simulink model "Manuever_3"  (R2023b)
settings: Solver=FixedStepAuto  StartTime=0.0  StopTime=50  RelTol=1e-3  EnableMultiTasking=on
libraries: legoev3lib x7
settings Model: ExtModeBatchMode=on  ExtModeTrigDuration=2  Creator=Krish  LastModifiedBy=Krish
settings SolverCC: PositivePriorityOrder=on  AutoInsertRateTranBlk=on
settings OptimizationCC: EnhancedBackFolding=on  PassReuseOutputArgsAs=Individual arguments  ZeroExternalMemoryAtStartup=off  ZeroInternalMemoryAtStartup=off  MaxStackSize=64  OptimizeBlockOrder=speed  DifferentSizesBufferReuse=on  OptimizationCustomize=off  EfficientTunableParamExpr=on
settings DebuggingCC: ParameterTunabilityLossMsg=error
settings HardwareCC: ProdBitPerPointer=32  ProdBitPerSizeT=32  ProdBitPerPtrDiffT=32  ProdLargestAtomicInteger=Long  ProdWordSize=32  ProdHWDeviceType=ARM Compatible->ARM 9
settings SFSimCC: MATLABDynamicMemAlloc=off
settings RTWCC: Description=Embedded Coder  SystemTargetFile=ert.tlc  HardwareBoard=LEGO MINDSTORMS EV3  TLCOptions="-aInlineSetEventsForThisBaseRateFcn=TLC_FALSE -aSuppressMultiTaskScheduler=TLC_FALSE  -aRateBasedStepFcn=0"  TemplateMakefile=ert_default_tmf  Toolchain=Sourcery G++ Lite v2009q3
settings CodeAppCC: ForceParamTrailComments=on  IgnoreCustomStorageClasses=off  OperatorAnnotations=on  SimulinkDataObjDesc=on  SFDataObjDesc=on  InsertBlockDesc=on
settings ERTTargetCC: SupportContinuousTime=on  SupportVariableSizeSignals=on  ExtModeTransport=2  ExtModeStaticAlloc=on  ExtModeMexFile=ext_xcp  ExtModeIntrfLevel=Level2 - Open

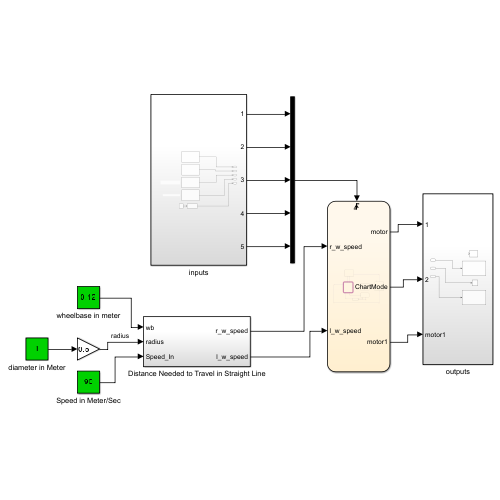
[thumbnail: Simulink's stored preview of the top-level diagram]
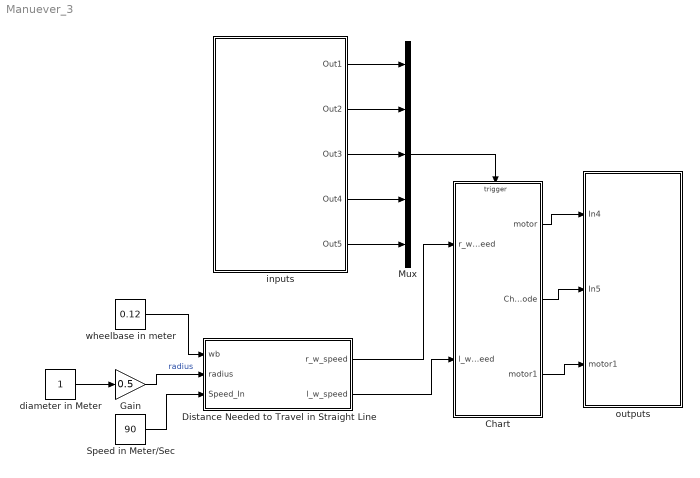
== system Manuever_3 ==
  Chart : Stateflow chart  TreatAsAtomicUnit=on
  Distance Needed to Travel in Straight Line : Subsystem
  Gain : Gain  Gain=0.5
  Mux : Mux  Inputs=5
  Speed in Meter/Sec : Constant  Value=90
  diameter in Meter : Constant
  inputs : Subsystem
  outputs : Subsystem
  wheelbase in meter : Constant  Value=0.12
  wires:
  Mux/1 -> Chart/Trigger
  inputs/1(Out1) -> Mux/1
  inputs/2(Out2) -> Mux/2
  inputs/3(Out3) -> Mux/3
  inputs/4(Out4) -> Mux/4
  inputs/5(Out5) -> Mux/5
  Chart/1(motor) -> outputs/1(In4)
  Chart/2(ChartMode) -> outputs/2(In5)
  Chart/3(motor1) -> outputs/3(motor1)
  Speed in Meter/Sec/1 -> Distance Needed to Travel in Straight Line/3(Speed_In)
  diameter in Meter/1 -> Gain/1
  Distance Needed to Travel in Straight Line/1(r_w_speed) -> Chart/1(r_w_speed)
  wheelbase in meter/1 -> Distance Needed to Travel in Straight Line/1(wb)
  Gain/1 -> Distance Needed to Travel in Straight Line/2(radius)  "radius"
  Distance Needed to Travel in Straight Line/2(l_w_speed) -> Chart/2(l_w_speed)

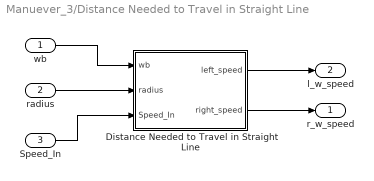
== system Manuever_3/Distance Needed to Travel in Straight Line ==
  wb : Inport
  radius : Inport  Port=2
  Speed_In : Inport  Port=3
  Distance Needed to Travel in Straight Line : Subsystem
  r_w_speed : Outport
  l_w_speed : Outport  Port=2
  wires:
  radius/1 -> Distance Needed to Travel in Straight Line/2(radius)
  Speed_In/1 -> Distance Needed to Travel in Straight Line/3(Speed_In)
  wb/1 -> Distance Needed to Travel in Straight Line/1(wb)
  Distance Needed to Travel in Straight Line/2(right_speed) -> r_w_speed/1
  Distance Needed to Travel in Straight Line/1(left_speed) -> l_w_speed/1

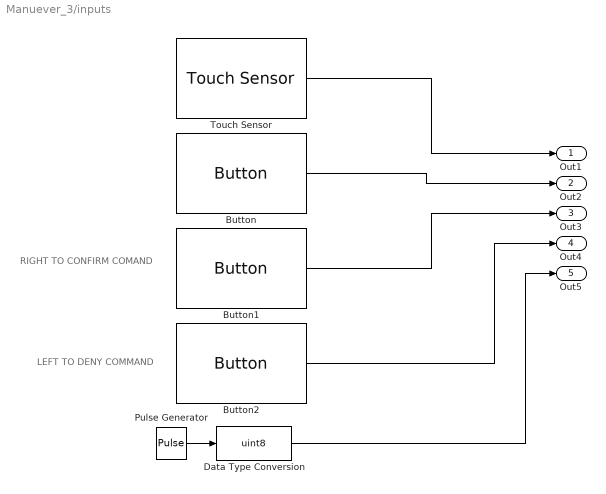
== system Manuever_3/inputs ==
  note: LEFT TO DENY COMMAND
  note: RIGHT TO CONFIRM COMAND
  Button : legoev3lib/Button  buttonType=Center  sampleTime=0.1
  Button1 : legoev3lib/Button  buttonType=Right  sampleTime=0.1
  Button2 : legoev3lib/Button  buttonType=Left  sampleTime=0.1
  Data Type Conversion : DataTypeConversion  OutDataTypeStr=uint8  SaturateOnIntegerOverflow=off  RndMeth=Floor
  Pulse Generator : DiscretePulseGenerator  Period=10  PulseWidth=5  SampleTime=0.1
  Touch Sensor : legoev3lib/Touch Sensor  portNumber=1  sampleTime=0.1
  Out1 : Outport
  Out2 : Outport  Port=2
  Out3 : Outport  Port=3
  Out4 : Outport  Port=4
  Out5 : Outport  Port=5
  wires:
  Pulse Generator/1 -> Data Type Conversion/1
  Button/1 -> Out2/1
  Button2/1 -> Out4/1
  Button1/1 -> Out3/1
  Data Type Conversion/1 -> Out5/1
  Touch Sensor/1 -> Out1/1

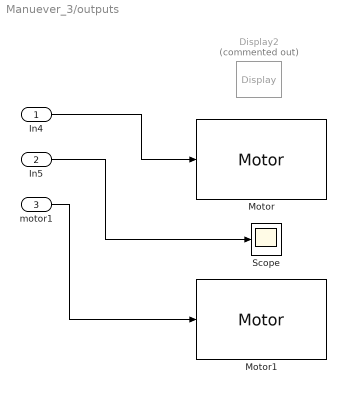
== system Manuever_3/outputs ==
  In4 : Inport
  In5 : Inport  Port=2
  motor1 : Inport  Port=3
  Display2 : legoev3lib/Display  Commented=on  slcdStr=Idle  slcdLine=1  slcdFormat=Decimal
  Motor : legoev3lib/Motor  sportNumber=A  sstopAction=Brake
  Motor1 : legoev3lib/Motor  sportNumber=B  sstopAction=Brake
  Scope : Scope
  wires:
  In4/1 -> Motor/1
  In5/1 -> Scope/1
  motor1/1 -> Motor1/1

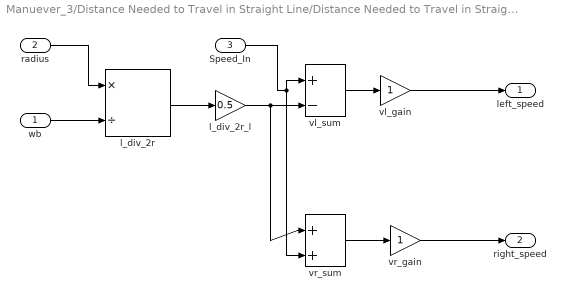
== system Manuever_3/Distance Needed to Travel in Straight Line/Distance Needed to Travel in Straight Line ==
  wb : Inport
  radius : Inport  Port=2
  Speed_In : Inport  Port=3
  l_div_2r : Product  Inputs=*/
  l_div_2r_l : Gain  Gain=0.5
  vl_gain : Gain
  vl_sum : Sum  Inputs=|+-
  vr_gain : Gain
  vr_sum : Sum  Inputs=|++
  left_speed : Outport
  right_speed : Outport  Port=2
  wires:
  radius/1 -> l_div_2r/1
  wb/1 -> l_div_2r/2
  l_div_2r/1 -> l_div_2r_l/1
  l_div_2r_l/1 -> vr_sum/1, vl_sum/2
  Speed_In/1 -> vr_sum/2, vl_sum/1
  vl_sum/1 -> vl_gain/1
  vr_sum/1 -> vr_gain/1
  vl_gain/1 -> left_speed/1
  vr_gain/1 -> right_speed/1

== stateflow chart Manuever_3/Chart ==
  settings: executeAtInitialization=1
  state TurnOffConfirm
    entry:
  state Off
    entry:
    motor=0;
    motor1=0;
    exit:
    turn_count=0;
  state On1
    entry:
    motor =r_w_speed;
    motor1=l_w_speed;
  state TurnOnConfirm
  state EmergencySTOP
    entry:
    motor=0;
    motor1=0;
  state mid_state
  TurnOffConfirm -> (junction 129) [order 2] : confirm
  (junction 129) -> Off
  TurnOffConfirm -> On1 [order 1] : deny
  On1 -> TurnOffConfirm [order 3] : Center_btn_pressed
  (default) -> Off
  On1 -> (junction 158) [order 2] : after(20,sec)
  (junction 158) -> (junction 142)
  TurnOnConfirm -> Off [order 2] : deny
  TurnOnConfirm -> On1 [order 1] : confirm
  Off -> TurnOnConfirm : Center_btn_pressed
  (junction 143) -> Off
  (junction 113) -> On1
  On1 -> (junction 115) [order 1]
  (junction 115) -> EmergencySTOP : e_btnPressed
  EmergencySTOP -> (junction 128)
  (junction 120) -> EmergencySTOP
  mid_state -> (junction 113) [order 2] : e_btnPressed
  (junction 128) -> mid_state : e_btnPressed
  mid_state -> (junction 120) [order 1] : after(4,sec)
  (junction 142) -> (junction 143) : after(50,sec)
  data: r_w_speed input; motor output =0; ChartMode output Enum: ChartModeType; motor1 output; turn_count local =0; l_w_speed input
  events: e_btnPressed input RISING_EDGE_EVENT; Center_btn_pressed input RISING_EDGE_EVENT; confirm input RISING_EDGE_EVENT; deny input RISING_EDGE_EVENT; clock input RISING_EDGE_EVENT
